simulink library "bes_and_inverter_PQ_command_block_lib_2011"  (Simulink 7.8)
settings: Solver=ode45  StartTime=0.0  StopTime=10.0  RelTol=1e-3
values from neighbouring files (symbols this model uses):
  C = IacRMS*18e-6    [BES_init.m]
  Iac_max = IGBT_currents(possible_currents(1))    [BES_init.m]
  L = Vdc_nom/(IacRMS*0.2/(2/fs))    [BES_init.m]
  Td_es_min = Ts    (= 8e-05)    [global_parameters.m]
  Vdc_max = IGBT_voltages(possible_voltages(1))    [BES_init.m]
libraries: battery_lib_2011 x1, Boost_rectifier_average_model_lib_2011 x1, simulink x1, Idq_controller_lib_2011 x1, PLL_three_phase_lib_2011 x1, dq_abc_lib_2011 x1, abc_dq_lib_2011 x1, windowed_limit_lib_2011 x1
settings Model: Creator=CH24070  LastModifiedBy=CH24070

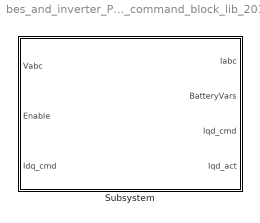
== system bes_and_inverter_PQ_command_block_lib_2011 ==
  Subsystem : Subsystem  mask(Battery Energy Storage System with AC inverter and Droop Control){max_power=1e6, batt_kWh=5000, VacRMS=480, Vdc_nom=1200}
      mask prompts: max_power "Peak Power (W)"; batt_kWh "Capacity (kWh)"; VacRMS "Grid Tie Line to Neutral Voltage (RMS)"; Vdc_nom "Nominal DC Battery Voltage"
      mask help: The block implements a battery energy storage system suitable for connecting to the grid. It responds to grid voltage changes by injecting current into the grid. The model is a non-switching average model.
      mask init:
      | global_parameters
      | BES_init
      mask Help:
      | This block will likely need a filter and transformer on it's output in order to connect to a high power line.
      | 
      | A unit delay block  on the Iabc output can help remove algebraic loops with minimal impact on simulation results.
      | 
      | 
      | Block Parameters:
      | Peak Power- Maximum power the unit can transfer.
      | Capacity- Amount of energy in the battery.
      | Grid Tie Line to Neutral Voltage- RMS voltage for the grid tie interface.
      | Nominal DC Battery Voltage- Open circuit full charge voltage.
      | Real Power Droop Gain- Ratio of Watts to Hz for injecting power to the grid in response to frequency changes.
      | Reactive Power Droop Gain- Ratio of kVars to RMS volts for injecting reactive power to the grid.
      | Droop Filter Cut Off- Fastest frequency that will be responded to for injecting power to the grid.
      | 
      | 
      | Block Connections:
      | Vabc- Grid voltage for each of the three phases.
      | Enable- Set to zero for no power.  Set to 1 to enable energy tranfer.
      | Iabc- Grid current for each of the three phases.  Connect to your grid.  Positive is into the grid.
      | Battery_vars- A vector of battery voltage, capacity, and current out of the battery.
      | Iqd_cmd- Commanded q and d axis currents.
      | Iqd_act- Actual q and d axis currents.
      mask Display:
      | image(imread('grid_storage_battery.jpg'))
      | color('white')
      | fprintf('%d kW Peak', max_power/1e3)
      | color('black')
      | port_label('input',1,'Vabc')
      | port_label('input',2,'Enable')
      | port_label('input',3,'Idq_cmd')
      | port_label('output',1,'Iabc')
      | port_label('output',2,'Battery_vars')
      | port_label('output',3,'Iqd_cmd')
      | port_label('output',4,'Iqd_act')

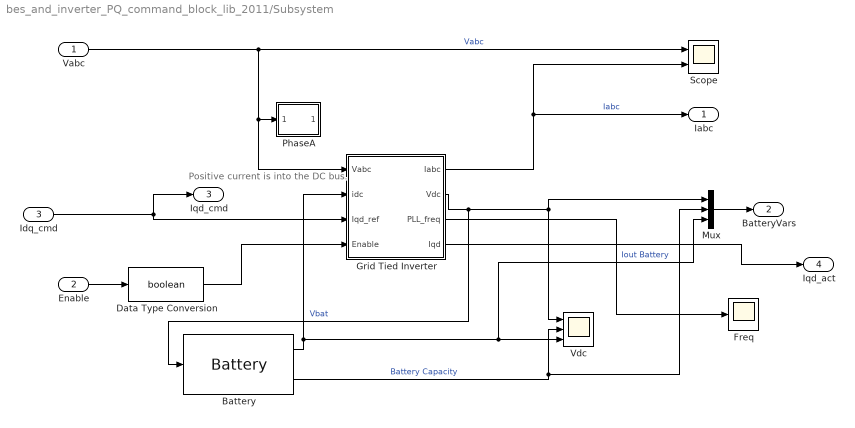
== system bes_and_inverter_PQ_command_block_lib_2011/Subsystem ==
  note: Positive current is into the DC bus.
  Vabc : Inport
  Enable : Inport  Port=2  OutDataTypeStr=double
  Idq_cmd : Inport  Port=3
  Battery : battery_lib_2011/Battery  energy=batt_kWh  esr=batt_esr  Vdc_nom=Vdc_nom
  Data Type Conversion : DataTypeConversion  OutDataTypeStr=boolean
  Freq : Scope
      settings: YMin=310  YMax=360
  Grid Tied Inverter : Subsystem
  Mux : Mux  Inputs=3
  PhaseA : Subsystem
  Scope : Scope  NumInputPorts=2
      settings: TimeRange=0.2  YMin=-550~-600  YMax=550~600  SaveName=ScopeData2
  Vdc : Scope  NumInputPorts=3
      settings: TimeRange=0.2  YMin=1200~0.735~-140  YMax=1214~0.8~0  SaveName=ScopeData3
  Iabc : Outport
  BatteryVars : Outport  Port=2
  Iqd_cmd : Outport  Port=3
  Iqd_act : Outport  Port=4
  wires:
  Vabc/1 -> Grid Tied Inverter/1(Vabc), PhaseA/1(In1), Scope/1  "Vabc"
  Grid Tied Inverter/2(Vdc) -> Battery/1, Vdc/1, Mux/1  "Vbat"
  Battery/1 -> Grid Tied Inverter/2(idc), Mux/3, Vdc/3  "Iout Battery"
  Battery/2 -> Mux/2, Vdc/2  "Battery Capacity"
  Grid Tied Inverter/1(Iabc) -> Iabc/1, Scope/2  "Iabc"
  Grid Tied Inverter/3(PLL_freq) -> Freq/1
  Mux/1 -> BatteryVars/1
  Grid Tied Inverter/4(Iqd) -> Iqd_act/1
  Idq_cmd/1 -> Grid Tied Inverter/3(Iqd_ref), Iqd_cmd/1
  Enable/1 -> Data Type Conversion/1
  Data Type Conversion/1 -> Grid Tied Inverter/4(Enable)

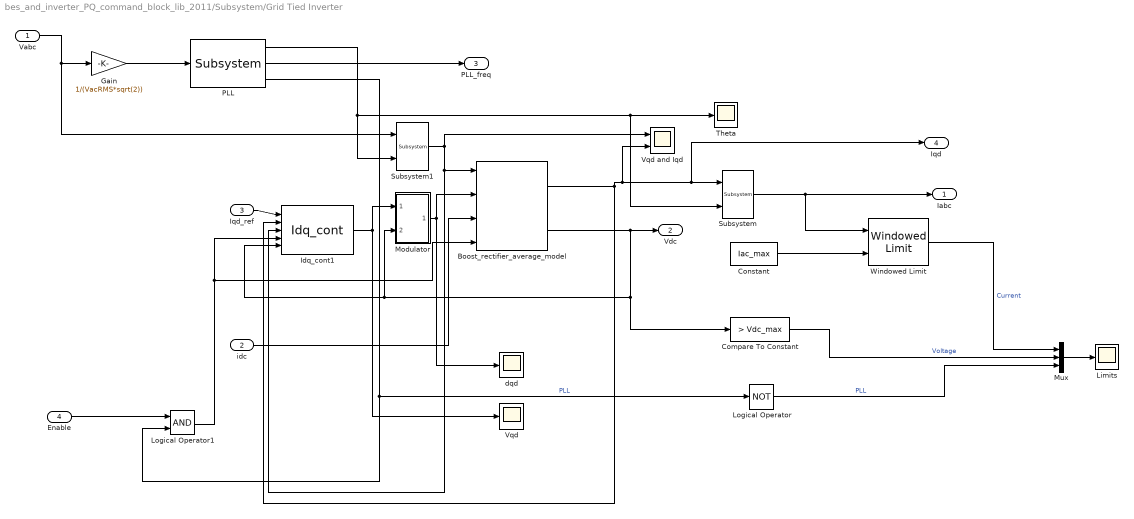
== system bes_and_inverter_PQ_command_block_lib_2011/Subsystem/Grid Tied Inverter ==
  Vabc : Inport
  idc : Inport  Port=2
  Iqd_ref : Inport  Port=3
  Enable : Inport  Port=4
  Boost_rectifier_average_model : Boost_rectifier_average_model_lib_2011/Boost_rectifier_average_model  C=C  L=L  Roff=Roff  Vdc_nom=Vdc_nom
  Compare To Constant : simulink/Logic and Bit Operations/Compare To Constant  relop=>  const=Vdc_max  OutDataTypeStr=boolean
  Constant : Constant  Value=Iac_max
  Gain : Gain  Gain=1/(VacRMS*sqrt(2))
  Idq_cont1 : Idq_controller_lib_2011/Idq_cont  L=L  iq_max=Iq_at_max  id_max=Id_at_max  kp=I_kp  ki=I_ki  Vdc_nom=Vdc_nom
  Limits : Scope
      settings: TimeRange=4.5  YMin=-1  YMax=2
  Logical Operator : Logic  Operator=NOT  AllPortsSameDT=off  OutDataTypeStr=boolean
  Logical Operator1 : Logic  AllPortsSameDT=off  OutDataTypeStr=boolean
  Modulator : Subsystem
  Mux : Mux  Inputs=3
  PLL : PLL_three_phase_lib_2011/Subsystem  PLL_Kp=PLL_Kp  PLL_Ki=PLL_Ki  PLL_freq_range=PLL_freq_range  PLL_lock_window=PLL_lock_window
  Subsystem : dq_abc_lib_2011/Subsystem
  Subsystem1 : abc_dq_lib_2011/Subsystem
  Theta : Scope
      settings: YMin=0  YMax=6.5  SaveName=ScopeData4
  Vqd : Scope
      settings: YMin=-2000  YMax=3500  SaveName=ScopeData7
  Vqd and Iqd : Scope  NumInputPorts=2
      settings: YMin=-800~-15  YMax=800~12.5  SaveName=ScopeData5
  Windowed Limit : windowed_limit_lib_2011/Windowed Limit
  dqd : Scope
      settings: YMin=-0.9409  YMax=-0.940825  SaveName=ScopeData6
  Iabc : Outport
  Vdc : Outport  Port=2
  PLL_freq : Outport  Port=3
  Iqd : Outport  Port=4
  wires:
  Vabc/1 -> Subsystem1/1, Gain/1
  Subsystem1/1 -> Vqd and Iqd/1, Idq_cont1/3, Boost_rectifier_average_model/1
  Boost_rectifier_average_model/1 -> Idq_cont1/2, Vqd and Iqd/2, Subsystem/1, Iqd/1
  Subsystem/1 -> Windowed Limit/1, Iabc/1
  Iqd_ref/1 -> Idq_cont1/1
  Idq_cont1/1 -> Vqd/1, Modulator/1(Vqd)
  PLL/1 -> Subsystem1/2, Subsystem/2, Theta/1
  idc/1 -> Boost_rectifier_average_model/3
  Boost_rectifier_average_model/2 -> Vdc/1, Idq_cont1/5, Modulator/2(Vdc), Compare To Constant/1
  Logical Operator1/1 -> Idq_cont1/4, Boost_rectifier_average_model/4
  Constant/1 -> Windowed Limit/2
  Windowed Limit/1 -> Mux/1  "Current"
  Compare To Constant/1 -> Mux/2  "Voltage"
  PLL/2 -> PLL_freq/1
  Modulator/1(dqd) -> Boost_rectifier_average_model/2, dqd/1
  PLL/3 -> Logical Operator/1, Logical Operator1/2  "PLL"
  Mux/1 -> Limits/1
  Logical Operator/1 -> Mux/3  "PLL"
  Gain/1 -> PLL/1
  Enable/1 -> Logical Operator1/1

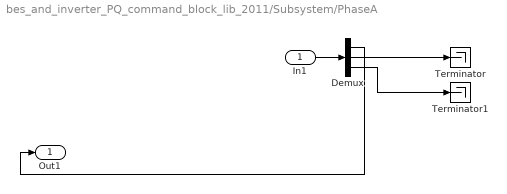
== system bes_and_inverter_PQ_command_block_lib_2011/Subsystem/PhaseA ==
  In1 : Inport
  Demux : Demux  Outputs=3
  Terminator : Terminator
  Terminator1 : Terminator
  Out1 : Outport
  wires:
  Demux/1 -> Out1/1
  In1/1 -> Demux/1
  Demux/3 -> Terminator1/1
  Demux/2 -> Terminator/1

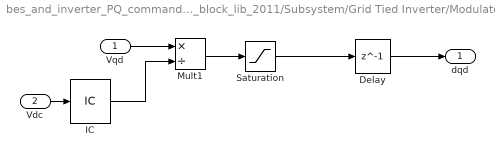
== system bes_and_inverter_PQ_command_block_lib_2011/Subsystem/Grid Tied Inverter/Modulator ==
  Vqd : Inport
  Vdc : Inport  Port=2
  Delay : Delay  DelayLength=1  InitialCondition=[0 0]  SampleTime=Td_es_min
  IC : InitialCondition  Value=Vdc_nom
  Mult1 : Product  Inputs=*/
  Saturation : Saturate  UpperLimit=1  LowerLimit=-1
  dqd : Outport
  wires:
  Mult1/1 -> Saturation/1
  Saturation/1 -> Delay/1
  Vqd/1 -> Mult1/1
  Vdc/1 -> IC/1
  IC/1 -> Mult1/2
  Delay/1 -> dqd/1
